simulink model "Control_Corriente_2021b"  (R2023b)
settings: Solver=FixedStepDiscrete  StartTime=0.0  StopTime=inf  FixedStep=0.001  RelTol=1e-3  EnableMultiTasking=on
libraries: arduinolib x20, simulink x6, arduinosensorlib x3
settings Model: ExtModeTrigDuration=2  Creator=leall  LastModifiedBy=marti
settings OptimizationCC: EnhancedBackFolding=on  PassReuseOutputArgsThreshold=0  MaxStackSize=64  OptimizeBlockOrder=speed  DifferentSizesBufferReuse=on  OptimizationCustomize=off
settings DebuggingCC: MultiTaskRateTransMsg=warning  ParameterTunabilityLossMsg=error  UnconnectedInputMsg=warning  UnconnectedOutputMsg=warning  UnconnectedLineMsg=warning
settings HardwareCC: ProdBitPerInt=16  ProdBitPerPointer=16  ProdBitPerSizeT=16  ProdBitPerPtrDiffT=16  ProdLargestAtomicFloat=None  ProdWordSize=8  ProdHWDeviceType=Atmel->AVR  UseEmbeddedCoderFeatures=off
settings ModelReferenceCC: EnableRefExpFcnMdlSchedulingChecks=on
settings SFSimCC: MATLABDynamicMemAlloc=off
settings RTWCC: Description=Embedded Coder  SystemTargetFile=ert.tlc  HardwareBoard=Arduino Mega 2560  TemplateMakefile=ert_default_tmf  Toolchain=Arduino AVR  BuildConfiguration=Faster Runs  DLArmComputeVersion=19.05
settings CodeAppCC: ForceParamTrailComments=on  OperatorAnnotations=on
settings ERTTargetCC: ERTCustomFileBanners=off  SupportContinuousTime=on  SupportNonInlinedSFcns=on  RemoveResetFunc=off  SupportVariableSizeSignals=on  ModelStepFunctionPrototypeControlCompliant=off  ExtModeTransport=3  ExtModeStaticAlloc=on  ExtModeStaticAllocSize=2048  ExtModeMexFile=ext_xcp  ExtModeIntrfLevel=Level2 - Open  ERTSrcFileBannerTemplate=codertarget_code_template.cgt  ERTHdrFileBannerTemplate=codertarget_code_template.cgt  ERTDataSrcFileTemplate=codertarget_code_template.cgt  ERTDataHdrFileTemplate=codertarget_code_template.cgt

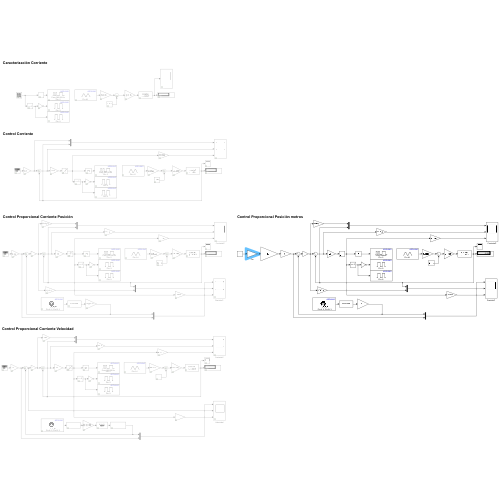
[thumbnail: Simulink's stored preview of the top-level diagram]
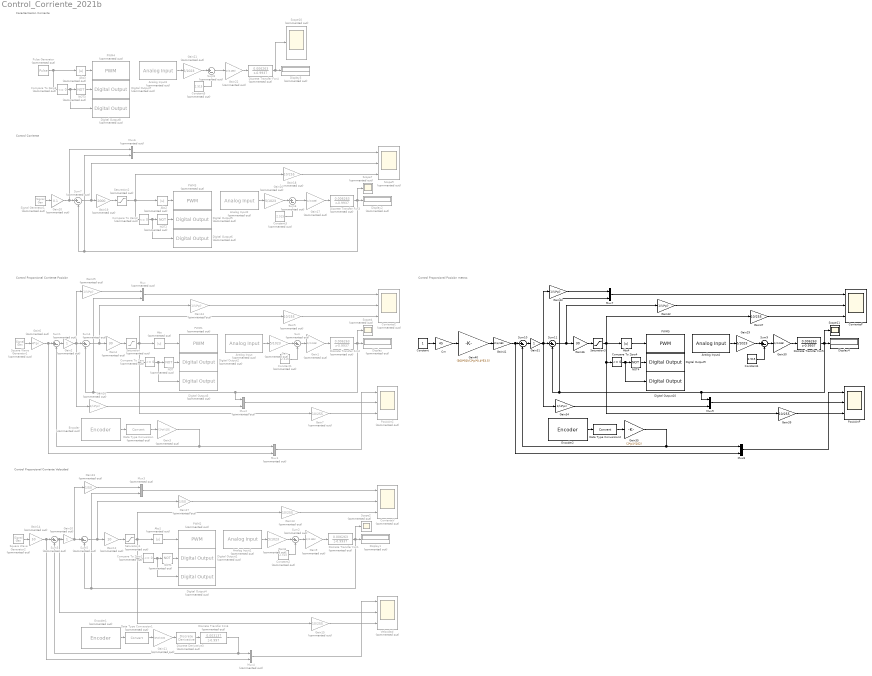
== system Control_Corriente_2021b ==
  note: Control Proporcional Corriente Posición
  note: Control Proporcional Corriente Velocidad
  note: Control Corriente
  note: Caracterización Corriente
  note: Control Proporcional Posición metros
  Abs{,1..3} (4 alike) : Abs  Commented=on  SaturateOnIntegerOverflow=off
  Abs4 : Abs  SaturateOnIntegerOverflow=off
  Analog Input{,1..3} (4 alike) : arduinolib/Analog Input  Commented=on  pinNumber=1  ReadResultsOnly=off  ConversionTriggerSource=Software  ExternalTriggerType=uint32( 0 )  OutputDataType=uint16  EnableConversionCompleteNotify=off  EnableOuputStatus=off  SampleTime=-1  blockPlatform=arduino
  Analog Input4 : arduinolib/Analog Input  pinNumber=1  ReadResultsOnly=off  ConversionTriggerSource=Software  ExternalTriggerType=uint32( 0 )  OutputDataType=uint16  EnableConversionCompleteNotify=off  EnableOuputStatus=off  SampleTime=-1  blockPlatform=arduino
  Cm : Gain  Gain=45
  Compare To Zero{,1..3} (4 alike) : simulink/Logic and Bit Operations/Compare To Zero  Commented=on  relop=<=  OutDataTypeStr=boolean
  Compare To Zero4 : simulink/Logic and Bit Operations/Compare To Zero  relop=<=  OutDataTypeStr=boolean
  Constant : Constant
  Constant{1..3,5} (4 alike) : Constant  Commented=on  Value=2.515
  Constant4 : Constant  Value=2.515
  CorrienteC : Scope  Commented=on  NumInputPorts=3
  CorrienteP : Scope  NumInputPorts=3
  CorrienteV : Scope  Commented=on  NumInputPorts=3
  Data Type Conversion : DataTypeConversion  Commented=on  SaturateOnIntegerOverflow=off  RndMeth=Floor
  Data Type Conversion1 : DataTypeConversion  Commented=on  SaturateOnIntegerOverflow=off  RndMeth=Floor
  Data Type Conversion2 : DataTypeConversion  SaturateOnIntegerOverflow=off  RndMeth=Floor
  Digital Output{1..2,5,7} (4 alike) : arduinolib/Digital Output  Commented=on  pinNumber=9  Direction=output  blockPlatform=arduino
  Digital Output10 : arduinolib/Digital Output  pinNumber=8  Direction=output  blockPlatform=arduino
  Digital Output{3..4,6,8} (4 alike) : arduinolib/Digital Output  Commented=on  pinNumber=8  Direction=output  blockPlatform=arduino
  Digital Output9 : arduinolib/Digital Output  pinNumber=9  Direction=output  blockPlatform=arduino
  Discrete Transfer Fcn{1..4} (4 alike) : DiscreteTransferFcn  Commented=on  Numerator=[0.006263]  Denominator=[1 -0.9937]
  Discrete Transfer Fcn5 : DiscreteTransferFcn  Numerator=[0.006263]  Denominator=[1 -0.9937]
  Discrete Transfer Fcn6 : DiscreteTransferFcn  Commented=on  Numerator=[0.003137]  Denominator=[1 -0.997]
  Discrete Derivative3 : simulink/Discrete/Discrete Derivative  Commented=on  gainval=1.0  ICPrevScaledInput=0.0  OutMin=[]  OutMax=[]  OutDataType=fixdt(1, 16)  OutScaling=2^-10  DoSatur=off
  Display{,1..3} (4 alike) : Display  Commented=on
  Display4 : Display
  Encoder : arduinosensorlib/Encoder  Commented=on  InputA=2  InputB=3  Mode=No reset  SampleTime=-1
  Encoder1 : arduinosensorlib/Encoder  Commented=on  InputA=2  InputB=3  Mode=No reset  SampleTime=-1
  Encoder2 : arduinosensorlib/Encoder  InputA=2  InputB=3  Mode=No reset  SampleTime=-1
  Gain{,8,16,21} (4 alike) : Gain  Commented=on  Gain=5/1023
  Gain{1,9,17,22} (4 alike) : Gain  Commented=on  Gain=1/(0.185)
  Gain10 : Gain  Commented=on
  Gain11 : Gain  Commented=on  Gain=(2*pi)/102
  Gain12 : Gain  Commented=on  Gain=10
  Gain{5,7,13,15,18} (5 alike) : Gain  Commented=on  Gain=10/255
  Gain14 : Gain  Commented=on  Gain=50
  Gain19 : Gain  Commented=on  Gain=2000
  Gain2 : Gain  Commented=on
  Gain20 : Gain  Commented=on  Gain=0.1
  Gain23 : Gain  Commented=on  Gain=1/50
  Gain24 : Gain  Commented=on  Gain=1/(4*pi)
  Gain25 : Gain  Commented=on  Gain=1/(4*pi)
  Gain26 : Gain  Commented=on  Gain=1/(4*pi)
  Gain27 : Gain  Commented=on  Gain=1/50
  Gain29 : Gain  Gain=5/1023
  Gain3 : Gain  Commented=on  Gain=(2*pi)/102
  Gain30 : Gain  Gain=1/(0.185)
  Gain31 : Gain
  Gain32 : Gain  Gain=1/(4*pi)
  Gain33 : Gain  Gain=1/(4*pi)
  Gain34 : Gain  Gain=1/(4*pi)
  Gain35 : Gain  Gain=(2*pi)/(102)
  Gain36 : Gain  Gain=30
  Gain37 : Gain  Gain=10/255
  Gain39 : Gain  Gain=10/255
  Gain4 : Gain  Commented=on  Gain=30
  Gain40 : Gain  Gain=(360*50)/(2*pi*0.4*53.5)
  Gain41 : Gain  Gain=2*pi/180
  Gain6 : Gain  Commented=on  Gain=4*pi
  Mux{,1..4,6} (6 alike) : Mux  Commented=on  Inputs=2
  Mux7 : Mux  Inputs=2
  Mux8 : Mux  Inputs=2
  Mux9 : Mux  Inputs=2
  NOT{,1..3} (4 alike) : Logic  Commented=on  Operator=NOT  IconShape=distinctive  AllPortsSameDT=off  OutDataTypeStr=boolean
  NOT4 : Logic  Operator=NOT  IconShape=distinctive  AllPortsSameDT=off  OutDataTypeStr=boolean
  PWM{1..4} (4 alike) : arduinolib/PWM  Commented=on  pinNumber=5  frequencyType=Specify  desiredFrequency=980.39  achievableFrequency=980.3922
  PWM5 : arduinolib/PWM  pinNumber=5  frequencyType=Default  desiredFrequency=980.39  achievableFrequency=980.3922
  PosiciónC : Scope  Commented=on  NumInputPorts=3
  PosiciónP : Scope  NumInputPorts=3
  Pulse Generator : DiscretePulseGenerator  Commented=on  PulseType=Time based  Amplitude=255  Period=10  PulseWidth=50
  Saturation : Saturate  Commented=on  UpperLimit=255  LowerLimit=-255
  Saturation1 : Saturate  Commented=on  UpperLimit=255  LowerLimit=-255
  Saturation2 : Saturate  Commented=on  UpperLimit=255  LowerLimit=-255
  Saturation3 : Saturate  UpperLimit=255  LowerLimit=-255
  Scope{2,4,7,10} (4 alike) : Scope  Commented=on
  Scope11 : Scope
  Scope9 : Scope  Commented=on  NumInputPorts=3
  Signal Generator1 : SignalGenerator  Commented=on  WaveForm=square  Frequency=0.1
  Square Wave Generator1 : SignalGenerator  Commented=on  WaveForm=square  Frequency=0.1
  Square Wave Generator2 : SignalGenerator  Commented=on  WaveForm=square  Frequency=0.1
  Sum{,1..8} (9 alike) : Sum  Commented=on  Inputs=|+-
  Sum10 : Sum  Inputs=|+-
  Sum11 : Sum  Inputs=|+-
  Sum9 : Sum  Inputs=|+-
  Velocidad : Scope  Commented=on  NumInputPorts=3
  wires:
  Compare To Zero/1 -> Digital Output3/1, NOT/1
  NOT/1 -> Digital Output2/1
  Abs/1 -> PWM1/1
  Encoder/1 -> Data Type Conversion/1
  Analog Input/1 -> Gain/1
  Constant1/1 -> Sum/2
  Gain/1 -> Sum/1
  Gain1/1 -> Discrete Transfer Fcn2/1
  Sum/1 -> Gain1/1
  Discrete Transfer Fcn2/1 -> Mux2/1, Sum4/2, Mux/2, Display/1, Scope4/1
  Gain4/1 -> Saturation/1
  Saturation/1 -> Compare To Zero/1, Gain7/1, Gain5/1, Abs/1
  Gain5/1 -> CorrienteC/3
  Mux/1 -> CorrienteC/1
  Sum1/1 -> Gain2/1
  Square Wave Generator1/1 -> Gain6/1
  Gain6/1 -> Mux1/2, Sum1/1
  Mux2/1 -> PosiciónC/2
  Gain3/1 -> Mux1/1, Sum1/2
  Data Type Conversion/1 -> Gain3/1
  Gain7/1 -> PosiciónC/3
  Gain15/1 -> Velocidad/3
  Mux4/1 -> Velocidad/1
  Square Wave Generator2/1 -> Gain14/1
  Data Type Conversion1/1 -> Gain11/1
  Sum2/1 -> Gain9/1
  Gain9/1 -> Discrete Transfer Fcn1/1
  Abs1/1 -> PWM2/1
  Encoder1/1 -> Data Type Conversion1/1
  Gain14/1 -> Mux4/2, Sum3/1
  Mux3/1 -> CorrienteV/1
  Gain13/1 -> CorrienteV/3
  Compare To Zero1/1 -> Digital Output4/1, NOT1/1
  Saturation1/1 -> Compare To Zero1/1, Gain15/1, Gain13/1, Abs1/1
  Discrete Transfer Fcn1/1 -> Sum5/2, Mux3/2, Display1/1, Scope2/1
  Gain10/1 -> Gain23/1, Sum5/1
  Sum3/1 -> Velocidad/2, Gain10/1
  Constant2/1 -> Sum2/2
  Sum5/1 -> Gain27/1, Gain12/1
  Analog Input1/1 -> Gain8/1
  Gain12/1 -> Saturation1/1
  Gain8/1 -> Sum2/1
  NOT1/1 -> Digital Output1/1
  Gain11/1 -> Discrete Derivative3/1
  Discrete Derivative3/1 -> Discrete Transfer Fcn6/1
  Discrete Transfer Fcn6/1 -> Sum3/2, Mux4/1
  Mux1/1 -> PosiciónC/1
  Sum6/1 -> Gain17/1
  Gain17/1 -> Discrete Transfer Fcn3/1
  Abs2/1 -> PWM3/1
  Mux6/1 -> Scope9/1
  Gain18/1 -> Scope9/3
  Compare To Zero2/1 -> Digital Output6/1, NOT2/1
  Analog Input2/1 -> Gain16/1
  Constant3/1 -> Sum6/2
  NOT2/1 -> Digital Output5/1
  Gain16/1 -> Sum6/1
  Sum7/1 -> Scope9/2, Gain19/1
  Signal Generator1/1 -> Gain20/1
  Gain19/1 -> Saturation2/1
  Discrete Transfer Fcn3/1 -> Sum7/2, Mux6/2, Scope7/1, Display2/1
  Gain20/1 -> Mux6/1, Sum7/1
  Saturation2/1 -> Gain18/1, Compare To Zero2/1, Abs2/1
  Pulse Generator/1 -> Compare To Zero3/1, Abs3/1
  Discrete Transfer Fcn4/1 -> Scope10/1, Display3/1
  Constant5/1 -> Sum8/2
  Abs3/1 -> PWM4/1
  NOT3/1 -> Digital Output7/1
  Analog Input3/1 -> Gain21/1
  Gain21/1 -> Sum8/1
  Gain22/1 -> Discrete Transfer Fcn4/1
  Compare To Zero3/1 -> Digital Output8/1, NOT3/1
  Sum8/1 -> Gain22/1
  Gain23/1 -> Mux3/1
  Sum4/1 -> Gain24/1, Gain4/1
  Gain24/1 -> CorrienteC/2
  Gain25/1 -> Mux/1
  Gain26/1 -> Mux2/2
  Gain27/1 -> CorrienteV/2
  Gain2/1 -> Gain25/1, Gain26/1, Sum4/1
  Gain34/1 -> Mux9/2
  Gain32/1 -> CorrienteP/2
  Gain39/1 -> PosiciónP/3
  Mux7/1 -> CorrienteP/1
  Gain35/1 -> Mux8/1, Sum10/2
  Data Type Conversion2/1 -> Gain35/1
  Gain37/1 -> CorrienteP/3
  Saturation3/1 -> Compare To Zero4/1, Gain39/1, Gain37/1, Abs4/1
  Gain30/1 -> Discrete Transfer Fcn5/1
  Discrete Transfer Fcn5/1 -> Mux9/1, Sum11/2, Mux7/2, Display4/1, Scope11/1
  Analog Input4/1 -> Gain29/1
  NOT4/1 -> Digital Output9/1
  Sum10/1 -> Gain31/1
  Constant4/1 -> Sum9/2
  Compare To Zero4/1 -> Digital Output10/1, NOT4/1
  Gain31/1 -> Gain33/1, Gain34/1, Sum11/1
  Mux9/1 -> PosiciónP/2
  Abs4/1 -> PWM5/1
  Sum9/1 -> Gain30/1
  Sum11/1 -> Gain32/1, Gain36/1
  Gain29/1 -> Sum9/1
  Gain33/1 -> Mux7/1
  Gain36/1 -> Saturation3/1
  Mux8/1 -> PosiciónP/1
  Encoder2/1 -> Data Type Conversion2/1
  Gain41/1 -> Mux8/2, Sum10/1
  Gain40/1 -> Gain41/1
  Constant/1 -> Cm/1
  Cm/1 -> Gain40/1
